simulink model "01_ee_a"  (R2023a)
settings: Solver=VariableStepDiscrete  StartTime=0.0  StopTime=6  RelTol=1e-3  EnableMultiTasking=on
PreLoadFcn:
  | %DFIG Data
  | clear;
  | NumberOfDFIG=100;
  | PnomDFIG=2e6*NumberOfDFIG; % Nominal power of DFIG(VA)
  | VnomDFIG=690;       % Line-Line voltage (Vrms)
  | fnom=50;
  | Rs=0.0108;     %pu
  | Lls=0.102;      %pu
  | Rr=0.01021;       %pu
  | Llr=0.11;      %pu
  | Lm=3.362;         %pu
  | Hg=2;         %Inertia constant (s)
  | F=0.01;         %Friction factor (pu)
  | p=2;            %Number of pairs of poles
  | kt=3;     %Rotor/Stator turns rotio
  | slip=-0.1;
  | 
  | %DC link
  | Vdc_nom=1200;       %Volts
  | C_DClink=15000e-6*NumberOfDFIG; %Farads
  | 
  | %Choke data
  | R_RL=0.15/100;  %pu
  | L_RL=0.15;      %pu
InitFcn:
  | Ts_Power = 10e-6;
  | Ts_Control = 100e-6;
  | PWM_freq=50*40;
undefined symbols (not defined in the file): D1, Delta, DiscIntNeverNeededParam
libraries: powerlib_extras x23, spsThreePhaseVIMeasurementLib x4, simulink_extras x4, spsThreePhaseTransformerTwoWindingsLib x2, spsUniversalBridgeLib x2, spsThreePhaseSeriesRLCBranchLib x2, spsParallelRLCBranchLib x1, spsThreePhaseProgrammableVoltageSourceLib x1, spsAsynchronousMachinepuUnitsLib x1, spsThreePhaseSeriesRLCLoadLib x1, spsGroundLib x1, spsMultimeterLib x1
(part 2 of 2)

== system 01_ee_a/Grid-side converter Control system/DC bus voltage Regulator/Discrete PI Controller ==
  note: Discrete PID Controller
  note: Pierre Giroux, Gilbert Sybille
      | Power System Simulation Laboratory
      | IREQ, Hydro-Quebc
  Error : Inport
  Discrete-Time Integrator : DiscreteIntegrator  InitialCondition=Init  SampleTime=Ts  LimitOutput=on  UpperSaturationLimit=UpperLimit  LowerSaturationLimit=LowerLimit  ICPrevOutput=DiscIntNeverNeededParam  ICPrevScaledInput=DiscIntNeverNeededParam
  Kp4 : Gain  Gain=Kp  SaturateOnIntegerOverflow=on  OutDataTypeStr=Inherit: Same as input  ParamDataTypeStr=Inherit: Same as input
  Kp5 : Gain  Gain=Ki  SaturateOnIntegerOverflow=on  OutDataTypeStr=Inherit: Same as input  ParamDataTypeStr=Inherit: Same as input
  Saturation2 : Saturate  UpperLimit=UpperLimit  LowerLimit=LowerLimit
  Scope : Scope  NumInputPorts=4
  Sum6 : Sum  InputSameDT=on  SaturateOnIntegerOverflow=on  OutDataTypeStr=Inherit: Same as first input
  Out : Outport  InitialOutput=0
  wires:
  Saturation2/1 -> Out/1, Scope/4
  Discrete-Time Integrator/1 -> Sum6/2, Scope/3
  Kp4/1 -> Sum6/1, Scope/2
  Kp5/1 -> Discrete-Time Integrator/1
  Sum6/1 -> Saturation2/1
  Error/1 -> Kp5/1, Kp4/1, Scope/1

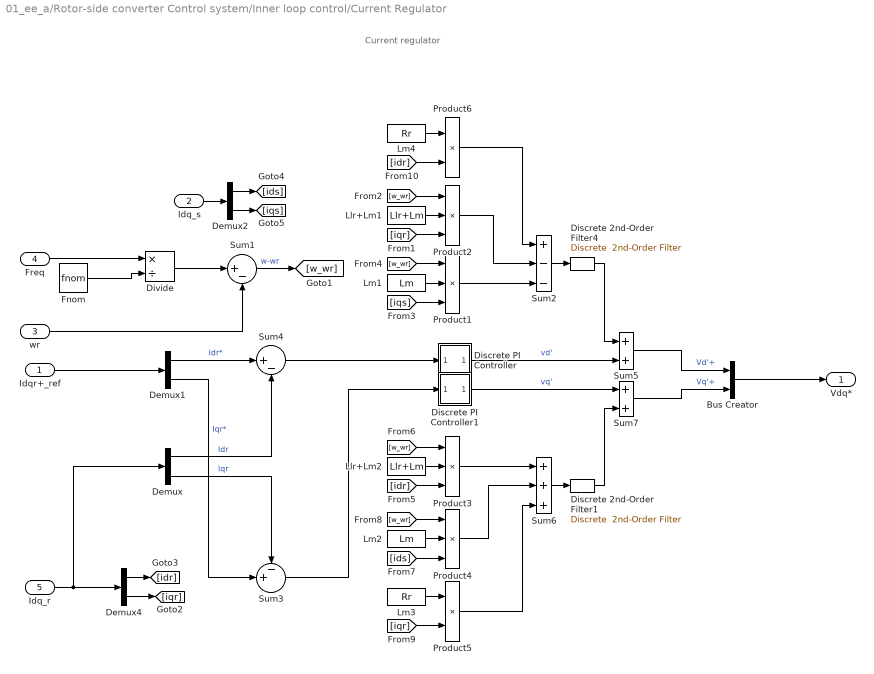
== system 01_ee_a/Rotor-side converter Control system/Inner loop control/Current Regulator ==
  note: Current regulator
  Idqr+_ref : Inport
  Idq_s : Inport  Port=2
  wr : Inport  Port=3
  Freq : Inport  Port=4
  Idq_r : Inport  Port=5
  Bus Creator : BusCreator  Inputs=2
  Demux{,1..2,4} (4 alike) : Demux  Outputs=2
      settings: DisplayOption=none
  Discrete PI Controller : Subsystem  AncestorBlock=|  DialogController=POWERSYS.PowerSysDialog  mask(Discrete PI Controller){Kp=Kp_rotor_side_cur_reg_P, Ki=Ki_rotor_side_cur_reg_P, Par_Limits=[Limit_U -Limit_U], Init=0, Ts=Ts_Control}
      | powerlib_extras/Discrete 
      | Control Blocks/Discrete
      | PI Controller
      mask prompts: Kp "Proportional gain (Kp):"; Ki "Integral gain (Ki):"; Par_Limits "Output limits: [ Upper   Lower ]"; Init "Output initial value:"; Ts "Sample time:"
      mask help: This block implements a discrete PI controller.
      mask init:
      | UpperLimit=Par_Limits(1);
      | LowerLimit=Par_Limits(2);
      | power_initmask();
      mask Help: This block is part of a subset of blocks in the Extras library that does not have documentation associated with it, other than the block mask description.
      mask Display: disp('PI');
  Discrete PI Controller1 : Subsystem  AncestorBlock=|  DialogController=POWERSYS.PowerSysDialog  mask(Discrete PI Controller){Kp=Kp_rotor_side_cur_reg_P, Ki=Ki_rotor_side_cur_reg_P, Par_Limits=[Limit_U -Limit_U], Init=0, Ts=Ts_Control}
      | powerlib_extras/Discrete 
      | Control Blocks/Discrete
      | PI Controller
      mask prompts: Kp "Proportional gain (Kp):"; Ki "Integral gain (Ki):"; Par_Limits "Output limits: [ Upper   Lower ]"; Init "Output initial value:"; Ts "Sample time:"
      mask help: This block implements a discrete PI controller.
      mask init:
      | UpperLimit=Par_Limits(1);
      | LowerLimit=Par_Limits(2);
      | power_initmask();
      mask Help: This block is part of a subset of blocks in the Extras library that does not have documentation associated with it, other than the block mask description.
      mask Display: disp('PI');
  Discrete 2nd-Order Filter1 : powerlib_extras/Discrete  Control Blocks/Discrete  2nd-Order Filter  FilterType=Lowpass  Fo=50  Zeta=0.707  Ts=Ts_Power  Initialize=off  Vac_Init=[0.8 -25 60]  Vdc_Init=-0.4  PlotResponse=off  param1=[1 5000 10]
  Discrete 2nd-Order Filter4 : powerlib_extras/Discrete  Control Blocks/Discrete  2nd-Order Filter  FilterType=Lowpass  Fo=50  Zeta=0.707  Ts=Ts_Power  Initialize=off  Vac_Init=[0.8 -25 60]  Vdc_Init=-0.4  PlotResponse=off  param1=[1 5000 10]
  Divide : Product  Inputs=*/
  Fnom : Constant  Value=fnom
  Llr+Lm1 : Constant  Value=Llr+Lm
  Llr+Lm2 : Constant  Value=Llr+Lm
  Lm1 : Constant  Value=Lm
  Lm2 : Constant  Value=Lm
  Lm3 : Constant  Value=Rr
  Lm4 : Constant  Value=Rr
  Product{1..4} (4 alike) : Product  Inputs=3  SaturateOnIntegerOverflow=on  OutDataTypeStr=Inherit: Same as first input
  Product5 : Product  SaturateOnIntegerOverflow=on  OutDataTypeStr=Inherit: Same as first input
  Product6 : Product  SaturateOnIntegerOverflow=on  OutDataTypeStr=Inherit: Same as first input
  Sum1 : Sum  Inputs=|+-  InputSameDT=on  SaturateOnIntegerOverflow=on  OutDataTypeStr=Inherit: Same as first input
  Sum2 : Sum  Inputs=+--  InputSameDT=on  SaturateOnIntegerOverflow=on  OutDataTypeStr=Inherit: Same as first input
  Sum3 : Sum  Inputs=-+|  InputSameDT=on  SaturateOnIntegerOverflow=on  OutDataTypeStr=Inherit: Same as first input
  Sum4 : Sum  Inputs=|+-  InputSameDT=on  SaturateOnIntegerOverflow=on  OutDataTypeStr=Inherit: Same as first input
  Sum5 : Sum  InputSameDT=on  SaturateOnIntegerOverflow=on  OutDataTypeStr=Inherit: Same as first input
  Sum6 : Sum  Inputs=+++  InputSameDT=on  SaturateOnIntegerOverflow=on  OutDataTypeStr=Inherit: Same as first input
  Sum7 : Sum  InputSameDT=on  SaturateOnIntegerOverflow=on  OutDataTypeStr=Inherit: Same as first input
  Vdq* : Outport
  wires:
  Sum4/1 -> Discrete PI Controller/1(Error)
  Sum3/1 -> Discrete PI Controller1/1(Error)
  Demux1/1 -> Sum4/1  "Idr*"
  Demux1/2 -> Sum3/2  "Iqr*"
  Idq_s/1 -> Demux2/1
  wr/1 -> Sum1/2
  Demux2/1 -> [ids]
  Demux2/2 -> [iqs]
  Sum1/1 -> [w_wr]  "w-wr"
  [w_wr] -> Product2/1
  Llr+Lm1/1 -> Product2/2
  [iqs] -> Product1/3
  [w_wr] -> Product1/1
  Lm1/1 -> Product1/2
  [w_wr] -> Product3/1
  Llr+Lm2/1 -> Product3/2
  [ids] -> Product4/3
  [w_wr] -> Product4/1
  Lm2/1 -> Product4/2
  Sum7/1 -> Bus Creator/2  "Vq'+"
  Bus Creator/1 -> Vdq*/1
  Product4/1 -> Sum6/2
  Lm3/1 -> Product5/1
  Lm4/1 -> Product6/1
  Product1/1 -> Sum2/3
  Idqr+_ref/1 -> Demux1/1
  Demux/1 -> Sum4/2  "Idr"
  Demux/2 -> Sum3/1  "Iqr"
  [idr] -> Product6/2
  [iqr] -> Product2/3
  [iqr] -> Product5/2
  [idr] -> Product3/3
  Product6/1 -> Sum2/1
  Product2/1 -> Sum2/2
  Product3/1 -> Sum6/1
  Product5/1 -> Sum6/3
  Sum2/1 -> Discrete 2nd-Order Filter4/1
  Sum5/1 -> Bus Creator/1  "Vd'+"
  Freq/1 -> Divide/1
  Fnom/1 -> Divide/2
  Discrete PI Controller/1(Out) -> Sum5/2  "vd'"
  Discrete PI Controller1/1(Out) -> Sum7/1  "vq'"
  Sum6/1 -> Discrete 2nd-Order Filter1/1
  Divide/1 -> Sum1/1
  Idq_r/1 -> Demux4/1, Demux/1
  Demux4/2 -> [iqr]
  Demux4/1 -> [idr]
  Discrete 2nd-Order Filter4/1 -> Sum5/1
  Discrete 2nd-Order Filter1/1 -> Sum7/2

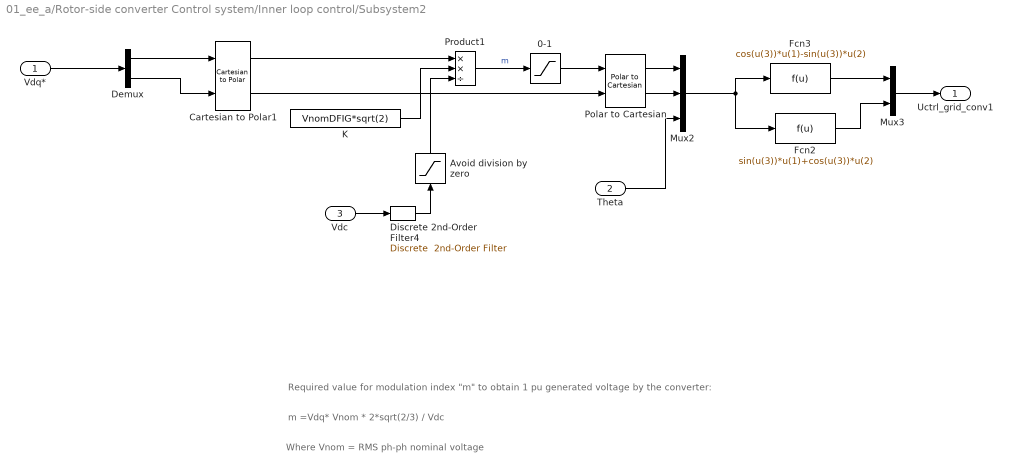
== system 01_ee_a/Rotor-side converter Control system/Inner loop control/Subsystem2 ==
  note: Required value for modulation index "m" to obtain 1 pu generated voltage by the converter:
  note: m =Vdq* Vnom * 2*sqrt(2/3) / Vdc
  note: Where Vnom = RMS ph-ph nominal voltage
  Vdq* : Inport
  Theta : Inport  Port=2
  Vdc : Inport  Port=3
  0-1 : Saturate  UpperLimit=1  LowerLimit=0
  Avoid division by zero : Saturate  UpperLimit=1e5  LowerLimit=10
  Cartesian to Polar1 : simulink_extras/Transformations/Cartesian to Polar
  Demux : Demux  Outputs=2
  Discrete 2nd-Order Filter4 : powerlib_extras/Discrete  Control Blocks/Discrete  2nd-Order Filter  FilterType=Lowpass  Fo=50  Zeta=0.707  Ts=Ts_Power  Initialize=off  Vac_Init=[0.8 -25 60]  Vdc_Init=-0.4  PlotResponse=off  param1=[1 5000 10]
  Fcn2 : Fcn  Expr=sin(u(3))*u(1)+cos(u(3))*u(2)  SampleTime=Ts_Power
  Fcn3 : Fcn  Expr=cos(u(3))*u(1)-sin(u(3))*u(2)  SampleTime=Ts_Power
  K : Constant  Value=VnomDFIG*sqrt(2)
  Mux2 : Mux  Inputs=3
  Mux3 : Mux  Inputs=2
  Polar to Cartesian : simulink_extras/Transformations/Polar to Cartesian
  Product1 : Product  Inputs=**/  InputSameDT=on  SaturateOnIntegerOverflow=on  OutDataTypeStr=Inherit: Same as first input
  Uctrl_grid_conv1 : Outport
  wires:
  Mux3/1 -> Uctrl_grid_conv1/1
  Fcn3/1 -> Mux3/1
  Fcn2/1 -> Mux3/2
  Demux/1 -> Cartesian to Polar1/1
  Demux/2 -> Cartesian to Polar1/2
  0-1/1 -> Polar to Cartesian/1
  Product1/1 -> 0-1/1  "m"
  Vdc/1 -> Discrete 2nd-Order Filter4/1
  K/1 -> Product1/2
  Avoid division by zero/1 -> Product1/3
  Cartesian to Polar1/1 -> Product1/1
  Cartesian to Polar1/2 -> Polar to Cartesian/2
  Vdq*/1 -> Demux/1
  Polar to Cartesian/1 -> Mux2/1
  Polar to Cartesian/2 -> Mux2/2
  Theta/1 -> Mux2/3
  Mux2/1 -> Fcn3/1, Fcn2/1
  Discrete 2nd-Order Filter4/1 -> Avoid division by zero/1

== system 01_ee_a/Rotor-side converter Control system/Outer loop control/Discrete PI Controller2 ==
  note: Discrete PID Controller
  note: Pierre Giroux, Gilbert Sybille
      | Power System Simulation Laboratory
      | IREQ, Hydro-Quebc
  Error : Inport
  Discrete-Time Integrator : DiscreteIntegrator  InitialCondition=Init  SampleTime=Ts  LimitOutput=on  UpperSaturationLimit=UpperLimit  LowerSaturationLimit=LowerLimit  ICPrevOutput=DiscIntNeverNeededParam  ICPrevScaledInput=DiscIntNeverNeededParam
  Kp4 : Gain  Gain=Kp  SaturateOnIntegerOverflow=on  OutDataTypeStr=Inherit: Same as input  ParamDataTypeStr=Inherit: Same as input
  Kp5 : Gain  Gain=Ki  SaturateOnIntegerOverflow=on  OutDataTypeStr=Inherit: Same as input  ParamDataTypeStr=Inherit: Same as input
  Saturation2 : Saturate  UpperLimit=UpperLimit  LowerLimit=LowerLimit
  Sum6 : Sum  InputSameDT=on  SaturateOnIntegerOverflow=on  OutDataTypeStr=Inherit: Same as first input
  Out : Outport  InitialOutput=0
  wires:
  Saturation2/1 -> Out/1
  Discrete-Time Integrator/1 -> Sum6/2
  Kp4/1 -> Sum6/1
  Kp5/1 -> Discrete-Time Integrator/1
  Sum6/1 -> Saturation2/1
  Error/1 -> Kp5/1, Kp4/1

== system 01_ee_a/Rotor-side converter Control system/Inner loop control/Current Regulator/Discrete PI Controller ==
  note: Discrete PID Controller
  note: Pierre Giroux, Gilbert Sybille
      | Power System Simulation Laboratory
      | IREQ, Hydro-Quebc
  Error : Inport
  Discrete-Time Integrator : DiscreteIntegrator  InitialCondition=Init  SampleTime=Ts  LimitOutput=on  UpperSaturationLimit=UpperLimit  LowerSaturationLimit=LowerLimit  ICPrevOutput=DiscIntNeverNeededParam  ICPrevScaledInput=DiscIntNeverNeededParam
  Kp4 : Gain  Gain=Kp  SaturateOnIntegerOverflow=on  OutDataTypeStr=Inherit: Same as input  ParamDataTypeStr=Inherit: Same as input
  Kp5 : Gain  Gain=Ki  SaturateOnIntegerOverflow=on  OutDataTypeStr=Inherit: Same as input  ParamDataTypeStr=Inherit: Same as input
  Saturation2 : Saturate  UpperLimit=UpperLimit  LowerLimit=LowerLimit
  Scope : Scope  NumInputPorts=4
  Sum6 : Sum  InputSameDT=on  SaturateOnIntegerOverflow=on  OutDataTypeStr=Inherit: Same as first input
  Out : Outport  InitialOutput=0
  wires:
  Saturation2/1 -> Scope/4, Out/1
  Discrete-Time Integrator/1 -> Scope/3, Sum6/2
  Kp4/1 -> Scope/2, Sum6/1
  Kp5/1 -> Discrete-Time Integrator/1
  Sum6/1 -> Saturation2/1
  Error/1 -> Scope/1, Kp5/1, Kp4/1

== system 01_ee_a/Rotor-side converter Control system/Inner loop control/Current Regulator/Discrete PI Controller1 ==
  note: Pierre Giroux, Gilbert Sybille
      | Power System Simulation Laboratory
      | IREQ, Hydro-Quebc
  note: Discrete PID Controller
  Error : Inport
  Discrete-Time Integrator : DiscreteIntegrator  InitialCondition=Init  SampleTime=Ts  LimitOutput=on  UpperSaturationLimit=UpperLimit  LowerSaturationLimit=LowerLimit  ICPrevOutput=DiscIntNeverNeededParam  ICPrevScaledInput=DiscIntNeverNeededParam
  Kp4 : Gain  Gain=Kp  SaturateOnIntegerOverflow=on  OutDataTypeStr=Inherit: Same as input  ParamDataTypeStr=Inherit: Same as input
  Kp5 : Gain  Gain=Ki  SaturateOnIntegerOverflow=on  OutDataTypeStr=Inherit: Same as input  ParamDataTypeStr=Inherit: Same as input
  Saturation2 : Saturate  UpperLimit=UpperLimit  LowerLimit=LowerLimit
  Sum6 : Sum  InputSameDT=on  SaturateOnIntegerOverflow=on  OutDataTypeStr=Inherit: Same as first input
  Out : Outport  InitialOutput=0
  wires:
  Error/1 -> Kp4/1, Kp5/1
  Sum6/1 -> Saturation2/1
  Kp5/1 -> Discrete-Time Integrator/1
  Kp4/1 -> Sum6/1
  Discrete-Time Integrator/1 -> Sum6/2
  Saturation2/1 -> Out/1
